simulink model "dc_dc_ac"  (R2018a)
settings: Solver=VariableStepDiscrete  StartTime=0.0  StopTime=0.0167  RelTol=1e-3
libraries: powerlib x35, re_lib x2, powerlib_meascontrol x1
settings Model: Creator=mwkane  LastModifiedBy=mwkane

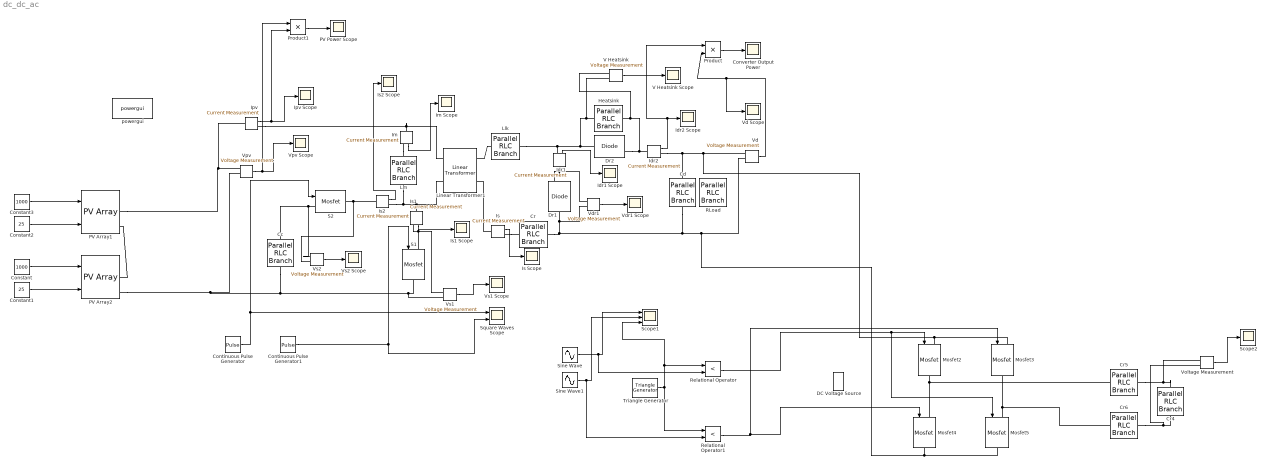
== system dc_dc_ac ==
  "Cc " : powerlib/Elements/Parallel RLC Branch  LConnTagsString=a  RConnTagsString=__new0  BranchType=C  Resistance=1  Inductance=1e-3  SetiL0=off  InitialCurrent=0  Capacitance=2.2e-06  Setx0=off  InitialVoltage=0  Measurements=None
  Cd : powerlib/Elements/Parallel RLC Branch  LConnTagsString=a  RConnTagsString=__new0  BranchType=C  Resistance=1  Inductance=1e-3  SetiL0=off  InitialCurrent=0  Capacitance=1e-6  Setx0=off  InitialVoltage=0  Measurements=None
  Constant : Constant  Value=1000
  Constant1 : Constant  Value=25
  Constant2 : Constant  Value=25
  Constant3 : Constant  Value=1000
  Continuous Pulse Generator : DiscretePulseGenerator  PulseType=Time based  Amplitude=5  Period=0.00002  PulseWidth=25
  Continuous Pulse Generator1 : DiscretePulseGenerator  PulseType=Time based  Amplitude=5  Period=0.00002  PulseWidth=75  PhaseDelay=0.000005
  Converter Output Power : Scope
  Cr : powerlib/Elements/Parallel RLC Branch  LConnTagsString=a  RConnTagsString=__new0  BranchType=C  Resistance=1  Inductance=1e-3  SetiL0=off  InitialCurrent=0  Capacitance=2.4e-6  Setx0=off  InitialVoltage=0  Measurements=None
  Cr4 : powerlib/Elements/Parallel RLC Branch  LConnTagsString=a  RConnTagsString=__new0  BranchType=R  Resistance=1e6  Inductance=2.6e-6  SetiL0=off  InitialCurrent=0  Capacitance=2.4e-6  Setx0=off  InitialVoltage=0  Measurements=None
  Cr5 : powerlib/Elements/Parallel RLC Branch  LConnTagsString=a  RConnTagsString=__new0  BranchType=L  Resistance=1  Inductance=15e-3  SetiL0=off  InitialCurrent=0  Capacitance=2.4e-6  Setx0=off  InitialVoltage=0  Measurements=None
  Cr6 : powerlib/Elements/Parallel RLC Branch  LConnTagsString=a  RConnTagsString=__new0  BranchType=L  Resistance=1  Inductance=15e-3  SetiL0=off  InitialCurrent=0  Capacitance=2.4e-6  Setx0=off  InitialVoltage=0  Measurements=None
  DC Voltage Source : powerlib/Electrical Sources/DC Voltage Source  Amplitude=100  Measurements=None
  Dr1 : powerlib/Power Electronics/Diode  Ron=0.01  Lon=0  Vf=0.8  IC=0  UseSnubber=0  Rs=inf  Cs=0  Measurements=on
  Dr2 : powerlib/Power Electronics/Diode  Ron=1  Lon=0  Vf=0.8  IC=0  UseSnubber=0  Rs=inf  Cs=0  Measurements=on
  Heatsink : powerlib/Elements/Parallel RLC Branch  LConnTagsString=a  RConnTagsString=__new0  BranchType=R  Resistance=1e3  Inductance=2.6e-6  SetiL0=off  InitialCurrent=0  Capacitance=2.4e-6  Setx0=off  InitialVoltage=0  Measurements=None
  Idr1 : powerlib/Measurements/Current Measurement  PhasorSimulation=off  OutputType=Complex  PSBequivalent=0
  Idr1 Scope : Scope
  Idr2 : powerlib/Measurements/Current Measurement  PhasorSimulation=off  OutputType=Complex  PSBequivalent=0
  Idr2 Scope : Scope
  Im : powerlib/Measurements/Current Measurement  PhasorSimulation=off  OutputType=Complex  PSBequivalent=0
  Im Scope : Scope
  "Ipv " : powerlib/Measurements/Current Measurement  PhasorSimulation=off  OutputType=Complex  PSBequivalent=0
  Ipv Scope : Scope
  Is : powerlib/Measurements/Current Measurement  PhasorSimulation=off  OutputType=Complex  PSBequivalent=0
  "Is Scope " : Scope
  Is1 : powerlib/Measurements/Current Measurement  PhasorSimulation=off  OutputType=Complex  PSBequivalent=0
  Is1 Scope : Scope
  "Is2 " : powerlib/Measurements/Current Measurement  PhasorSimulation=off  OutputType=Complex  PSBequivalent=0
  Is2 Scope : Scope
  Linear Transformer1 : powerlib/Elements/Linear Transformer  UNITS=SI  NominalPower=[ 25 100e3 ]  winding1=[9 0 0]  winding2=[38 0 0]  ThreeWindings=off  winding3=[3.15e+05 3.969e+07 6316.9]  RmLm=[1e6 0]  Measurements=Magnetization current  DataType=on
  Llk : powerlib/Elements/Parallel RLC Branch  LConnTagsString=a  RConnTagsString=__new0  BranchType=L  Resistance=1  Inductance=2.6e-6  SetiL0=off  InitialCurrent=0  Capacitance=2.4e-6  Setx0=off  InitialVoltage=0  Measurements=None
  Lm : powerlib/Elements/Parallel RLC Branch  LConnTagsString=a  RConnTagsString=__new0  BranchType=L  Resistance=1  Inductance=20e-6  SetiL0=off  InitialCurrent=0  Capacitance=2.4e-6  Setx0=off  InitialVoltage=0  Measurements=None
  Mosfet{2..5} (4 alike) : powerlib/Power Electronics/Mosfet  Ron=1.4  Lon=0  Rd=0.0000001  Vfd=1.5  IC=0  Rs=1e6  Cs=inf  Measurements=off
  PV Array1 : re_lib/Solar/PV Array  Npar=1  Nser=1  PlotType=array @ 25 deg.C & specified irradiances  S_vec="[ 1000  500  100 ]"  Temp_C_vec="[ 45 25  ]"  ModuleName=User-defined  PlotWhenSelected=off  Pm=179.9805  Ncell=36  Voc=24.06  Isc=9.77  Vm=19.67  Im=9.15  beta_Voc_pc=-0.28  alpha_Isc_pc=+0.04  beta_Voc=-0.067368  alpha_Isc=0.003908  IL=9.8911  I0=1.3829e-11  nI=0.95443  Rsh=60.4787  Rs=0.18212  BAL=off  Tc=1e-6  Tfilter=5e-5
  PV Array2 : re_lib/Solar/PV Array  Npar=1  Nser=1  PlotType=array @ 25 deg.C & specified irradiances  S_vec="[ 1000  500  100 ]"  Temp_C_vec="[ 45 25  ]"  ModuleName=User-defined  PlotWhenSelected=off  Pm=179.9805  Ncell=36  Voc=24.06  Isc=9.77  Vm=19.67  Im=9.15  beta_Voc_pc=-0.28  alpha_Isc_pc=+0.04  beta_Voc=-0.067368  alpha_Isc=0.003908  IL=9.8911  I0=1.3829e-11  nI=0.95443  Rsh=60.4787  Rs=0.18212  BAL=off  Tc=1e-6  Tfilter=5e-5
  PV Power Scope : Scope
  Product : Product
  Product1 : Product
  RLoad : powerlib/Elements/Parallel RLC Branch  LConnTagsString=a  RConnTagsString=__new0  BranchType=R  Resistance=1e3  Inductance=2.6e-6  SetiL0=off  InitialCurrent=0  Capacitance=2.4e-6  Setx0=off  InitialVoltage=0  Measurements=None
  Relational Operator : RelationalOperator  Operator=<  OutDataTypeStr=boolean  RndMeth=Simplest
  Relational Operator1 : RelationalOperator  Operator=<  OutDataTypeStr=boolean  RndMeth=Simplest
  S1 : powerlib/Power Electronics/Mosfet  Ron=5.6e-3  Lon=0  Rd=0.01  Vfd=0  IC=0  Rs=1e6  Cs=inf  Measurements=off
  S2 : powerlib/Power Electronics/Mosfet  Ron=5.6e-3  Lon=0  Rd=0.01  Vfd=0  IC=0  Rs=1e5  Cs=inf  Measurements=off
  Scope1 : Scope  NumInputPorts=3
  Scope2 : Scope
  Sine Wave : Sin  Frequency=60*2*pi  SampleTime=0
  Sine Wave1 : Sin  Frequency=60*2*pi  Phase=pi  SampleTime=0
  Square Waves Scope : Scope  NumInputPorts=2
  Triangle Generator : powerlib_meascontrol/Pulse & Signal Generators/Triangle Generator  Freq=16e3  Phase=0  Ts=0
  V Heatsink : powerlib/Measurements/Voltage Measurement  PhasorSimulation=off  OutputType=Complex  PSBequivalent=0
  V Heatsink Scope : Scope
  Vd : powerlib/Measurements/Voltage Measurement  PhasorSimulation=off  OutputType=Complex  PSBequivalent=0
  Vd Scope : Scope
  Vdr1 : powerlib/Measurements/Voltage Measurement  PhasorSimulation=off  OutputType=Complex  PSBequivalent=0
  Vdr1 Scope : Scope
  Voltage Measurement : powerlib/Measurements/Voltage Measurement  PhasorSimulation=off  OutputType=Complex  PSBequivalent=0
  Vpv : powerlib/Measurements/Voltage Measurement  PhasorSimulation=off  OutputType=Complex  PSBequivalent=0
  Vpv Scope : Scope
  Vs1 : powerlib/Measurements/Voltage Measurement  PhasorSimulation=off  OutputType=Complex  PSBequivalent=0
  Vs1 Scope : Scope
  Vs2 : powerlib/Measurements/Voltage Measurement  PhasorSimulation=off  OutputType=Complex  PSBequivalent=0
  Vs2 Scope : Scope
  powergui : powerlib/powergui  Priority=1  SimulationMode=Discrete  SampleTime=50e-10  frequency=60  Iterations=50  frequencyindice=0  Pbase=100e6  ErrMax=1e-4  UnitsV=kV  UnitsW=MW  buscounter=0  FunctionMessages=off  echomessages=off  EnableUseOfTLC=off  CurrentSourceSwitches=off  DisableSnubberDevices=off  DisableRonSwitches=off  DisableVfSwitches=off  DisplayEquations=off  SolverType=Tustin/Backward Euler (TBE)  Interpol=off  ExternalGateDelay=off  methode=off  Ts=100  x0status=blocks  SPID=on  SwTol=0  HookPort=off  RestoreLinks=warning  ResistiveCurrentMeasurement=off  Frange=[0:2:500]  Ylog=off  Xlog=on  ShowGrid=off  save=off  variable=ZData  structure=0  ZoomFFT=off  StartTime=0.0  cycles=1  DisplayStyle=1  fundamental=60  FreqAxis=off  MaxFrequency=1000  frequencyindicesteady=1  RmsSteady=1  display=off
  wires:
  Constant/1 -> PV Array2/1
  Constant1/1 -> PV Array2/2
  "Ipv "/1 -> Product1/2, Ipv Scope/1
  Vpv/1 -> Product1/1, Vpv Scope/1
  Vd/1 -> Product/2, Vd Scope/1
  Continuous Pulse Generator/1 -> S2/1, Square Waves Scope/1
  Continuous Pulse Generator1/1 -> S1/1, Square Waves Scope/2
  Im/1 -> Im Scope/1
  Vs1/1 -> Vs1 Scope/1
  Vs2/1 -> Vs2 Scope/1
  "Is2 "/1 -> Is2 Scope/1
  Is1/1 -> Is1 Scope/1
  V Heatsink/1 -> V Heatsink Scope/1
  Idr1/1 -> Idr1 Scope/1
  Vdr1/1 -> Vdr1 Scope/1
  Idr2/1 -> Product/1, Idr2 Scope/1
  Is/1 -> "Is Scope "/1
  Product/1 -> Converter Output Power/1
  Product1/1 -> PV Power Scope/1
  Constant2/1 -> PV Array1/2
  Constant3/1 -> PV Array1/1
  Sine Wave1/1 -> Relational Operator1/2, Scope1/2
  Relational Operator1/1 -> Mosfet4/1, Mosfet3/1
  Voltage Measurement/1 -> Scope2/1
  Sine Wave/1 -> Relational Operator/2, Scope1/1
  Relational Operator/1 -> Mosfet5/1, Mosfet2/1
  Triangle Generator/1 -> Relational Operator1/1, Scope1/3, Relational Operator/1
  connections:
  Vpv/LConn1 -- PV Array1/RConn1 -- "Ipv "/LConn1
  Dr2/LConn1 -- Heatsink/LConn1 -- V Heatsink/LConn2 -- Idr1/RConn1 -- Llk/RConn1
  "Ipv "/RConn1 -- Im/LConn1 -- Linear Transformer1/LConn1
  S1/LConn1 -- Is1/RConn1 -- Vs1/LConn1
  Vpv/LConn2 -- PV Array2/RConn2 -- "Cc "/RConn1 -- S1/RConn1 -- Vs1/LConn2
  Linear Transformer1/RConn1 -- Llk/LConn1
  S2/LConn1 -- Vs2/LConn1 -- "Cc "/LConn1
  Im/RConn1 -- Lm/LConn1
  S2/RConn1 -- "Is2 "/LConn1 -- Vs2/LConn2
  Lm/RConn1 -- Is1/LConn1 -- Linear Transformer1/LConn2 -- "Is2 "/RConn1
  Dr2/RConn1 -- Heatsink/RConn1 -- V Heatsink/LConn1 -- Idr2/LConn1
  Vdr1/LConn1 -- Idr1/LConn1 -- Dr1/RConn1
  Is/RConn1 -- Cr/LConn1
  Is/LConn1 -- Linear Transformer1/RConn2
  PV Array2/RConn1 -- PV Array1/RConn2
  Vd/LConn1 -- Mosfet3/LConn1 -- Mosfet2/LConn1 -- Idr2/RConn1 -- Cd/LConn1
  Cr4/RConn1 -- Cr6/RConn1 -- Voltage Measurement/LConn2
  Cr4/LConn1 -- Cr5/RConn1 -- Voltage Measurement/LConn1
  Mosfet3/RConn1 -- Cr6/LConn1 -- Mosfet5/LConn1
  Cr/RConn1 -- Mosfet5/RConn1 -- Mosfet4/RConn1 -- Vd/LConn2 -- Cd/RConn1 -- Vdr1/LConn2 -- Dr1/LConn1
  Cr5/LConn1 -- Mosfet2/RConn1 -- Mosfet4/LConn1
